simulink model "V1_Matlab_Function_Block_Model"  (R2017a)
settings: Solver=ode45  StartTime=0.0  StopTime=10  MaxStep=0.01  RelTol=1e-3  EnableMultiTasking=on
values from neighbouring files (symbols this model uses):
  g = 9.81    [Modell.m]    (also in sFunModell.m = block.DialogPrm(1).Data)
  l1 = 0.2    [Modell.m]    (also in sFunModell.m = block.DialogPrm(4).Data)
  l2 = 0.2    [Modell.m]    (also in sFunModell.m = block.DialogPrm(5).Data)
  m1 = 0.3    [Modell.m]    (also in sFunModell.m = block.DialogPrm(2).Data)
  m2 = 0.3    [Modell.m]    (also in sFunModell.m = block.DialogPrm(3).Data)
  Rp1 = 1e-2    (= 0.01)    [Modell.m]    (also in sFunModell.m = block.DialogPrm(6).Data)
  Rp2 = 1e-3    (= 0.001)    [Modell.m]    (also in sFunModell.m = block.DialogPrm(7).Data)
settings Model: Creator=ajentsch  LastModifiedBy=Ali Kerem Sacakli
settings DataIOCC: LimitDataPoints=on
settings OptimizationCC: LifeSpan=inf
settings DebuggingCC: AllowSymbolicDim=off  SFUnexpectedBacktrackingDiag=warning  SFNoUnconditionalDefaultTransitionDiag=warning  SFExecutionAtInitializationDiag=none
settings ModelReferenceCC: PropagateSignalLabelsOutOfModel=off
settings GRTTargetCC: TargetLangStandard=C89/C90 (ANSI)
settings ConfigComp: CovMetricSettings=dw  CovHtmlReporting=on  CovSaveCumulativeToWorkspaceVar=on  CovSaveSingleToWorkspaceVar=on  CovExternalEMLEnable=off

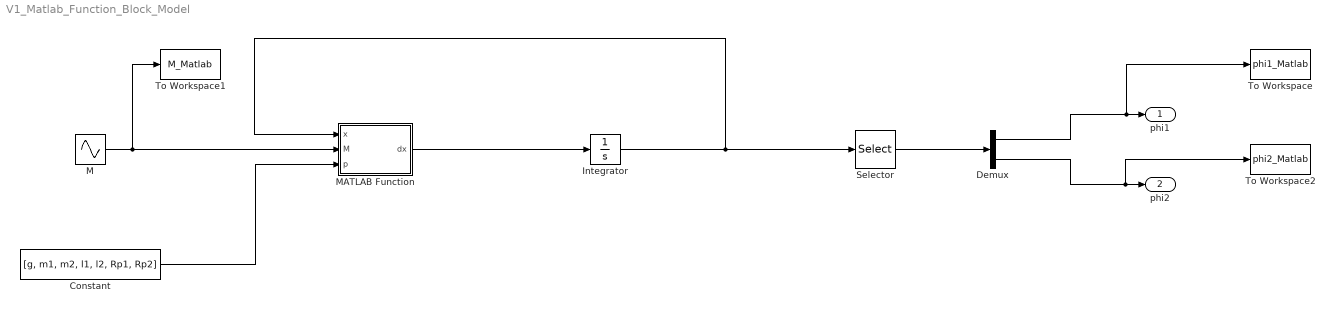
== system V1_Matlab_Function_Block_Model ==
  Constant : Constant  Value=[g, m1, m2, l1, l2, Rp1, Rp2]
  Demux : Demux  Outputs=2
  Integrator : Integrator
  M : Sin  Amplitude=0.1  SampleTime=0
  MATLAB Function : MATLAB Function  TreatAsAtomicUnit=on
  Selector : Selector  InputPortWidth=4  IndexOptions=Index vector (dialog)  Indices=[1 3]  OutputSizes=1
  To Workspace : ToWorkspace  VariableName=phi1_Matlab  SaveFormat=Timeseries  SampleTime=-1
  To Workspace1 : ToWorkspace  VariableName=M_Matlab  SaveFormat=Timeseries  SampleTime=-1
  To Workspace2 : ToWorkspace  VariableName=phi2_Matlab  SaveFormat=Timeseries  SampleTime=-1
  phi1 : Outport
  phi2 : Outport  Port=2
  wires:
  Demux/2 -> To Workspace2/1, phi2/1
  Demux/1 -> To Workspace/1, phi1/1
  Selector/1 -> Demux/1
  Constant/1 -> MATLAB Function/3(p)
  M/1 -> To Workspace1/1, MATLAB Function/2(M)
  MATLAB Function/1(dx) -> Integrator/1
  Integrator/1 -> MATLAB Function/1(x), Selector/1

== matlab function V1_Matlab_Function_Block_Model/MATLAB Function ==
  data: x input; dx output; M input; p input
function dx = fcn(x,M,p)
%#codegen

% Zustände definieren
phi1  = x(1);
dphi1 = x(2);
phi2  = x(3);
dphi2 = x(4);

% Parameter definieren
g = p(1);
m1 = p(2);
m2 = p(3);
l1 = p(4);
l2 = p(5);
Rp1 = p(6);
Rp2 = p(7);

% Bewegungsgleichungen des Modells
ddphi1 = -(6*(4*Rp1*dphi1*l2 - 4*M*l2 + 6*Rp2*dphi1*l1*cos(phi1 - phi2) - 6*Rp2*dphi2*l1*cos(phi1 - phi2) + (3*g*l1*l2*m2*sin(phi1 - 2*phi2))/2 + (3*dphi1^2*l1^2*l2*m2*sin(2*phi1 - 2*phi2))/2 + 2*dphi2^2*l1*l2^2*m2*sin(phi1 - phi2) + 2*g*l1*l2*m1*sin(phi1) + (5*g*l1*l2*m2*sin(phi1))/2))/(l1^2*l2*(8*m1 + 15*m2 - 9*m2*cos(2*phi1 - 2*phi2)));

ddphi2 = (6*(4*Rp2*dphi1*l1*m1 - 6*M*l2*m2*cos(phi1 - phi2) + 12*Rp2*dphi1*l1*m2 - 4*Rp2*dphi2*l1*m1 - 12*Rp2*dphi2*l1*m2 + 6*dphi1^2*l1^2*l2*m2^2*sin(phi1 - phi2) - 3*g*l1*l2*m2^2*sin(phi2) + (3*dphi2^2*l1*l2^2*m2^2*sin(2*phi1 - 2*phi2))/2 + 3*g*l1*l2*m2^2*sin(2*phi1 - phi2) + 6*Rp1*dphi1*l2*m2*cos(phi1 - phi2) + 2*dphi1^2*l1^2*l2*m1*m2*sin(phi1 - phi2) - (g*l1*l2*m1*m2*sin(phi2))/2 + (3*g*l1*l2*m1*m2*sin(2*phi1 - phi2))/2))/(l1*l2^2*m2*(8*m1 + 15*m2 - 9*m2*cos(2*phi1 - 2*phi2)));

% Zustandsraummodell
dx = [dphi1; ddphi1; dphi2; ddphi2];
